simulink model "n2_linearized_system_control"  (R2023b)
settings: Solver=VariableStepAuto  StartTime=0.0  StopTime=3  RelTol=1e-3
values from neighbouring files (symbols this model uses):
  Alin = [0    -k/Jl + m*g*l*sin(x2_bar)/Jl                     0           k/Jl ... (first row only)    [collaborative_class_main.m]    (also in n0_collaborative_class_main.m)
  Blin = [0; 0; 1/Jm; 0]    [collaborative_class_main.m]    (also in n0_collaborative_class_main.m)
  dx_0 = [0;1;0;1]*0.1    [n0_collaborative_class_main.m]    (also in svc_robot.m)
  K = place(Alin, Blin, p)    [collaborative_class_main.m]    (also in n0_collaborative_class_main.m)
  K_H2_V = K_H2(:, 5)    [collaborative_class_main.m]    (also in n0_collaborative_class_main.m)
  K_H2_X = K_H2(:,1:4)    [collaborative_class_main.m]    (also in n0_collaborative_class_main.m)
  K_lqeta = K_lqe(:, 5)    [collaborative_class_main.m]    (also in n0_collaborative_class_main.m)
  K_lqx = K_lqe(:,1:4)    [collaborative_class_main.m]    (also in n0_collaborative_class_main.m)
  Kv = -K_ext(1, 5)    [collaborative_class_main.m]    (also in n0_collaborative_class_main.m)
  Kx = -K_ext(1, 1:4)    [collaborative_class_main.m]    (also in n0_collaborative_class_main.m)
  u_bar = m*g*l*cos(x2_bar)    [collaborative_class_main.m]    (also in n0_collaborative_class_main.m; svc_robot.m)
undefined symbols (not defined in the file or in its folder): K_lq
settings Model: Creator=teoma  LastModifiedBy=teoma

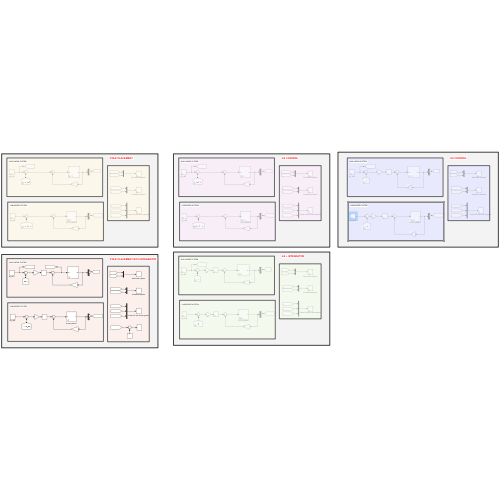
[thumbnail: Simulink's stored preview of the top-level diagram]
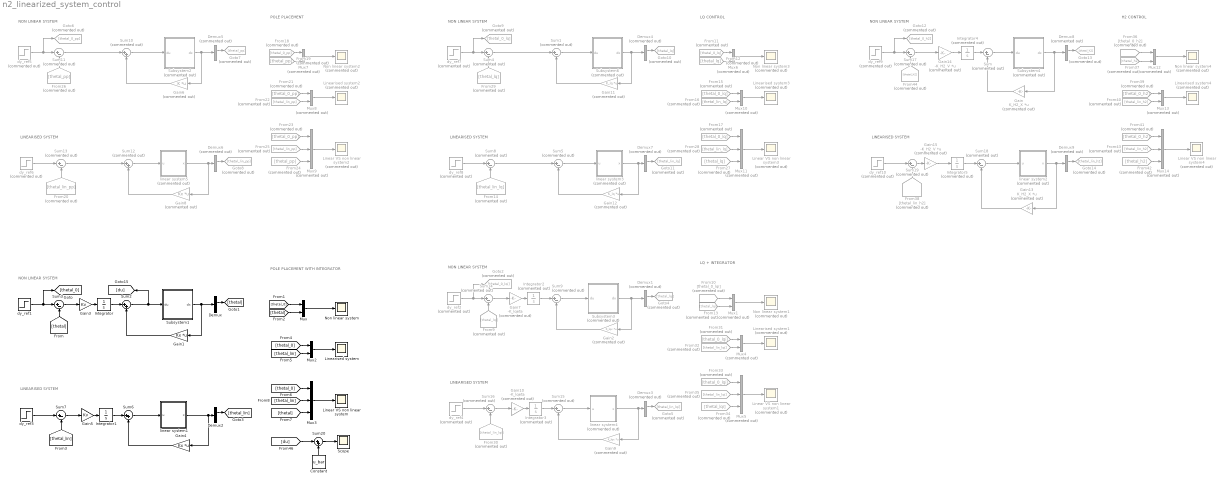
== system n2_linearized_system_control ==
  note: POLE PLACEMENT WITH INTEGRATOR
  note: NON LINEAR SYSTEM
  note: LINEARISED SYSTEM
  note: POLE PLACEMENT
  note: LINEARISED SYSTEM
  note: NON LINEAR SYSTEM
  note: NON LINEAR SYSTEM
  note: LQ CONTROL
  note: LINEARISED SYSTEM
  note: NON LINEAR SYSTEM
  note: LINEARISED SYSTEM
  note: LQ + INTEGRATOR
  note: LINEARISED SYSTEM
  note: H2 CONTROL
  note: NON LINEAR SYSTEM
  Constant : Constant  Value=u_bar
  Demux : Demux
  Demux{1,3..9} (8 alike) : Demux  Commented=on
  Demux2 : Demux
  From10 : From  Commented=on  GotoTag=thetal_0_lqi
  From11 : From  Commented=on  GotoTag=thetal_0_lq
  From12 : From  Commented=on  GotoTag=thetal_lq
  From13 : From  Commented=on  GotoTag=thetal_lqi
  From14 : From  Commented=on  GotoTag=thetal_lin_lq
  From15 : From  Commented=on  GotoTag=thetal_0_lq
  From16 : From  Commented=on  GotoTag=thetal_lin_lq
  From17 : From  Commented=on  GotoTag=thetal_0_lq
  From18 : From  Commented=on  GotoTag=thetal_0_pp
  From19 : From  Commented=on  GotoTag=thetal_pp
  From20 : From  Commented=on  GotoTag=thetal_lin_pp
  From21 : From  Commented=on  GotoTag=thetal_0_pp
  From22 : From  Commented=on  GotoTag=thetal_lin_pp
  From23 : From  Commented=on  GotoTag=thetal_0_pp
  From24 : From  Commented=on  GotoTag=thetal_pp
  From25 : From  Commented=on  GotoTag=thetal_lin_pp
  From26 : From  Commented=on  GotoTag=thetal_pp
  From27 : From  Commented=on  GotoTag=thetal_lq
  From28 : From  Commented=on  GotoTag=thetal_lin_lq
  From29 : From  Commented=on  GotoTag=thetal_lq
  From30 : From  Commented=on  GotoTag=thetal_lin_lqi
  From31 : From  Commented=on  GotoTag=thetal_0_lqi
  From32 : From  Commented=on  GotoTag=thetal_lin_lqi
  From33 : From  Commented=on  GotoTag=thetal_0_lqi
  From34 : From  Commented=on  GotoTag=thetal_lqi
  From35 : From  Commented=on  GotoTag=thetal_lin_lqi
  From36 : From  Commented=on  GotoTag=thetal_0_h2
  From37 : From  Commented=on  GotoTag=thetal_h2
  From38 : From  Commented=on  GotoTag=thetal_lin_h2
  From39 : From  Commented=on  GotoTag=thetal_0_h2
  From40 : From  Commented=on  GotoTag=thetal_lin_h2
  From41 : From  Commented=on  GotoTag=thetal_0_h2
  From42 : From  Commented=on  GotoTag=thetal_h2
  From43 : From  Commented=on  GotoTag=thetal_lin_h2
  From44 : From  Commented=on  GotoTag=thetal_h2
  From9 : From  Commented=on  GotoTag=thetal_lqi
  Gain : Gain  Commented=on  Gain=K_H2_X  Multiplication=Matrix(K*u) (u vector)
  Gain1 : Gain  Gain=Kx  Multiplication=Matrix(K*u) (u vector)
  Gain10 : Gain  Commented=on  Gain=-K_lqeta
  Gain11 : Gain  Commented=on  Gain=K_lq  Multiplication=Matrix(K*u) (u vector)
  Gain12 : Gain  Commented=on  Gain=K_lq  Multiplication=Matrix(K*u) (u vector)
  Gain13 : Gain  Commented=on  Gain=K_H2_X  Multiplication=Matrix(K*u) (u vector)
  Gain14 : Gain  Commented=on  Gain=-K_H2_V  Multiplication=Matrix(K*u) (u vector)
  Gain15 : Gain  Commented=on  Gain=-K_H2_V  Multiplication=Matrix(K*u) (u vector)
  Gain2 : Gain  Commented=on  Gain=K_lqx  Multiplication=Matrix(K*u) (u vector)
  Gain3 : Gain  Gain=Kv
  Gain4 : Gain  Gain=Kx  Multiplication=Matrix(K*u) (u vector)
  Gain5 : Gain  Gain=Kv
  Gain6 : Gain  Commented=on  Gain=K  Multiplication=Matrix(K*u) (u vector)
  Gain7 : Gain  Commented=on  Gain=-K_lqeta
  Gain8 : Gain  Commented=on  Gain=Kx  Multiplication=Matrix(K*u) (u vector)
  Gain9 : Gain  Commented=on  Gain=K_lqx  Multiplication=Matrix(K*u) (u vector)
  Goto10 : Goto  Commented=on  GotoTag=thetal_lq
  Goto11 : Goto  Commented=on  GotoTag=thetal_lin_lq
  Goto12 : Goto  Commented=on  GotoTag=thetal_0_h2
  Goto13 : Goto  Commented=on  GotoTag=thetal_h2
  Goto14 : Goto  Commented=on  GotoTag=thetal_lin_h2
  Goto2 : Goto  Commented=on  GotoTag=thetal_0_lqi
  Goto4 : Goto  Commented=on  GotoTag=thetal_lqi
  Goto5 : Goto  Commented=on  GotoTag=thetal_lin_lqi
  Goto6 : Goto  Commented=on  GotoTag=thetal_0_pp
  Goto7 : Goto  Commented=on  GotoTag=thetal_pp
  Goto8 : Goto  Commented=on  GotoTag=thetal_lin_pp
  Goto9 : Goto  Commented=on  GotoTag=thetal_0_lq
  Integrator : Integrator
  Integrator1 : Integrator
  Integrator{2..5} (4 alike) : Integrator  Commented=on
  Linear VS non linear system : Scope
  Linear VS non linear system{1..4} (4 alike) : Scope  Commented=on
  Linearised system : Scope
  Linearised system{1..4} (4 alike) : Scope  Commented=on
  Mux : Mux  Inputs=2
  Mux{1,4,6..8,10,12..13} (8 alike) : Mux  Commented=on  Inputs=2
  Mux{5,9,11,14} (4 alike) : Mux  Commented=on  Inputs=3
  Mux2 : Mux  Inputs=2
  Mux3 : Mux  Inputs=3
  Non linear system : Scope
  Non linear system{1..4} (4 alike) : Scope  Commented=on
  Scope : Scope
  Subsystem1 : Subsystem  mask{dx_0=dx_0}
      mask prompts: dx_0 "initial state"
  Subsystem2 : Subsystem  Commented=on  mask{dx_0=dx_0}
      mask prompts: dx_0 "initial state"
  Subsystem3 : Subsystem  Commented=on  mask{dx_0=dx_0}
      mask prompts: dx_0 "initial state"
  Subsystem4 : Subsystem  Commented=on  mask{dx_0=dx_0}
      mask prompts: dx_0 "initial state"
  Subsystem6 : Subsystem  Commented=on  mask{dx_0=dx_0}
      mask prompts: dx_0 "initial state"
  Sum{,1,4..5,8..9,11,13..19} (14 alike) : Sum  Commented=on  Inputs=|+-
  Sum10 : Sum  Commented=on  Inputs=|++
  Sum12 : Sum  Commented=on  Inputs=|++
  Sum2 : Sum  Inputs=|++
  Sum20 : Sum  Inputs=|++
  Sum3 : Sum  Inputs=|+-
  Sum6 : Sum  Inputs=|++
  Sum7 : Sum  Inputs=|+-
  dy_ref1 : Step  After=0.1  SampleTime=0
  dy_ref{2,4,9..10} (4 alike) : Step  Commented=on  Time=0  After=0.1  SampleTime=0
  dy_ref3 : Step  After=0.1  SampleTime=0
  dy_ref{5..8} (4 alike) : Step  Commented=on  After=0.1  SampleTime=0
  linear system1 : Subsystem  mask{dx_0=dx_0}
      mask prompts: dx_0 "initial state"
  linear system2 : Subsystem  Commented=on  mask{dx_0=dx_0}
      mask prompts: dx_0 "initial state"
  linear system3 : Subsystem  Commented=on  mask{dx_0=dx_0}
      mask prompts: dx_0 "initial state"
  linear system4 : Subsystem  Commented=on  mask{dx_0=dx_0}
      mask prompts: dx_0 "initial state"
  linear system5 : Subsystem  Commented=on  mask{dx_0=dx_0}
      mask prompts: dx_0 "initial state"
  wires:
  Subsystem1/1(dx) -> Gain1/1, Demux/1
  Sum2/1 -> [du], Subsystem1/1(du)
  Gain1/1 -> Sum2/2
  dy_ref1/1 -> [thetal_0], Sum3/1
  Mux/1 -> Non linear system/1
  Sum3/1 -> Gain3/1
  Gain3/1 -> Integrator/1
  Integrator/1 -> Sum2/1
  Demux/2 -> [thetal]
  [thetal] -> Sum3/2
  [thetal_0] -> Mux/1
  [thetal] -> Mux/2
  dy_ref3/1 -> Sum7/1
  Sum7/1 -> Gain5/1
  Sum6/1 -> linear system1/1(u)
  [thetal_lin] -> Mux2/2
  Gain4/1 -> Sum6/2
  Mux2/1 -> Linearised system/1
  Gain5/1 -> Integrator1/1
  Integrator1/1 -> Sum6/1
  [thetal_0] -> Mux2/1
  [thetal_lin] -> Sum7/2
  Demux2/2 -> [thetal_lin]
  linear system1/1(x) -> Gain4/1, Demux2/1
  [thetal_0] -> Mux3/1
  [thetal] -> Mux3/3
  [thetal_lin] -> Mux3/2
  Mux3/1 -> Linear VS non linear system/1
  Sum10/1 -> Subsystem2/1(du)
  Mux7/1 -> Non linear system2/1
  From21/1 -> Mux8/1
  From19/1 -> Mux7/2
  Gain6/1 -> Sum10/2
  Subsystem2/1(dx) -> Gain6/1, Demux5/1
  From23/1 -> Mux9/1
  Mux8/1 -> Linearised system2/1
  linear system5/1(x) -> Gain8/1, Demux6/1
  Demux5/2 -> Goto7/1
  From26/1 -> Sum11/2
  From18/1 -> Mux7/1
  Gain8/1 -> Sum12/2
  Demux6/2 -> Goto8/1
  From20/1 -> Sum13/2
  Mux9/1 -> Linear VS non linear system2/1
  dy_ref6/1 -> Sum13/1
  From22/1 -> Mux8/2
  From25/1 -> Mux9/2
  From24/1 -> Mux9/3
  dy_ref5/1 -> Goto6/1, Sum11/1
  Sum11/1 -> Sum10/1
  Sum13/1 -> Sum12/1
  From33/1 -> Mux5/1
  Sum8/1 -> Sum5/1
  From29/1 -> Sum4/2
  Subsystem6/1(dx) -> Gain11/1, Demux4/1
  Integrator3/1 -> Sum15/1
  From17/1 -> Mux11/1
  Sum1/1 -> Subsystem6/1(du)
  Mux1/1 -> Non linear system1/1
  From32/1 -> Mux4/2
  Mux10/1 -> Linearised system3/1
  Demux3/2 -> Goto5/1
  Demux7/2 -> Goto11/1
  From15/1 -> Mux10/1
  Demux1/2 -> Goto4/1
  Mux6/1 -> Non linear system3/1
  From14/1 -> Sum8/2
  From11/1 -> Mux6/1
  From27/1 -> Mux11/3
  Sum4/1 -> Sum1/1
  From31/1 -> Mux4/1
  Gain11/1 -> Sum1/2
  Sum15/1 -> linear system4/1(u)
  dy_ref2/1 -> Goto2/1, Sum14/1
  Gain7/1 -> Integrator2/1
  Gain2/1 -> Sum9/2
  From10/1 -> Mux1/1
  From12/1 -> Mux6/2
  Gain9/1 -> Sum15/2
  dy_ref4/1 -> Sum16/1
  Subsystem3/1(dx) -> Gain2/1, Demux1/1
  From35/1 -> Mux5/2
  Gain10/1 -> Integrator3/1
  Sum16/1 -> Gain10/1
  Sum5/1 -> linear system3/1(u)
  From9/1 -> Sum14/2
  dy_ref8/1 -> Sum8/1
  From13/1 -> Mux1/2
  linear system4/1(x) -> Gain9/1, Demux3/1
  Sum14/1 -> Gain7/1
  dy_ref7/1 -> Goto9/1, Sum4/1
  Mux4/1 -> Linearised system1/1
  Mux11/1 -> Linear VS non linear system3/1
  linear system3/1(x) -> Gain12/1, Demux7/1
  From16/1 -> Mux10/2
  From28/1 -> Mux11/2
  Sum9/1 -> Subsystem3/1(du)
  Mux5/1 -> Linear VS non linear system1/1
  Demux4/2 -> Goto10/1
  From30/1 -> Sum16/2
  Gain12/1 -> Sum5/2
  From34/1 -> Mux5/3
  Integrator2/1 -> Sum9/1
  From40/1 -> Mux13/2
  Demux9/2 -> Goto14/1
  From43/1 -> Mux14/2
  From38/1 -> Sum19/2
  From37/1 -> Mux12/2
  Mux12/1 -> Non linear system4/1
  From44/1 -> Sum17/2
  From42/1 -> Mux14/3
  dy_ref10/1 -> Sum19/1
  From36/1 -> Mux12/1
  Demux8/2 -> Goto13/1
  From39/1 -> Mux13/1
  Subsystem4/1(dx) -> Gain/1, Demux8/1
  dy_ref9/1 -> Goto12/1, Sum17/1
  From41/1 -> Mux14/1
  Mux14/1 -> Linear VS non linear system4/1
  linear system2/1(x) -> Gain13/1, Demux9/1
  Mux13/1 -> Linearised system4/1
  Gain/1 -> Sum/2
  Sum/1 -> Subsystem4/1(du)
  Sum18/1 -> linear system2/1(u)
  Gain13/1 -> Sum18/2
  Gain14/1 -> Integrator4/1
  Gain15/1 -> Integrator5/1
  Sum17/1 -> Gain14/1
  Integrator4/1 -> Sum/1
  Sum19/1 -> Gain15/1
  Integrator5/1 -> Sum18/1
  Sum20/1 -> Scope/1
  Constant/1 -> Sum20/2
  [du] -> Sum20/1
  Sum12/1 -> linear system5/1(u)

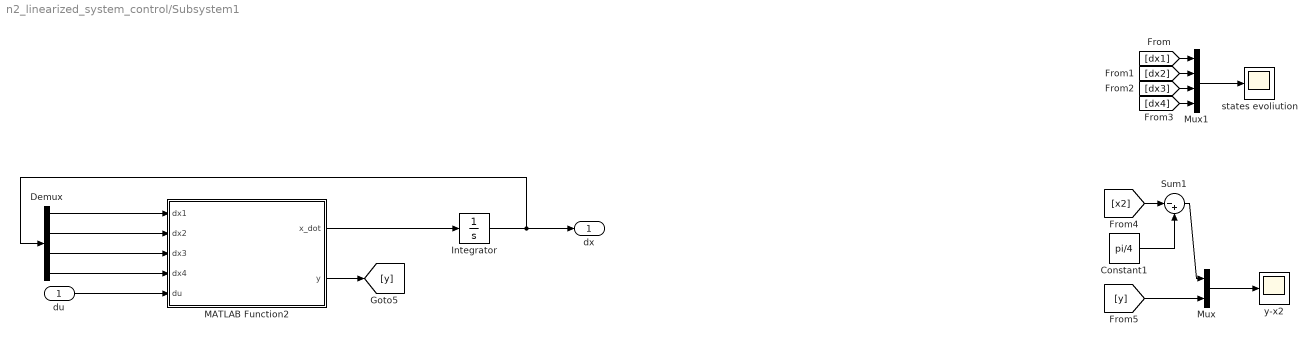
== system n2_linearized_system_control/Subsystem1 ==
  du : Inport
  Constant1 : Constant  Value=pi/4
  Demux : Demux
  Integrator : Integrator  InitialCondition=dx_0
  MATLAB Function2 : MATLAB Function  TreatAsAtomicUnit=on
  Mux : Mux  Inputs=2
  Mux1 : Mux
  Sum1 : Sum  Inputs=|-+
  "states evoliution " : Scope
  y-x2 : Scope
  dx : Outport
  wires:
  du/1 -> MATLAB Function2/5(du)
  MATLAB Function2/2(y) -> [y]
  Demux/1 -> MATLAB Function2/1(dx1)
  Demux/2 -> MATLAB Function2/2(dx2)
  Demux/3 -> MATLAB Function2/3(dx3)
  Demux/4 -> MATLAB Function2/4(dx4)
  MATLAB Function2/1(x_dot) -> Integrator/1
  Integrator/1 -> dx/1, Demux/1
  Mux/1 -> y-x2/1
  Sum1/1 -> Mux/1
  Constant1/1 -> Sum1/2
  [dx1] -> Mux1/1
  [dx2] -> Mux1/2
  [dx3] -> Mux1/3
  [dx4] -> Mux1/4
  Mux1/1 -> "states evoliution "/1
  [x2] -> Sum1/1
  [y] -> Mux/2

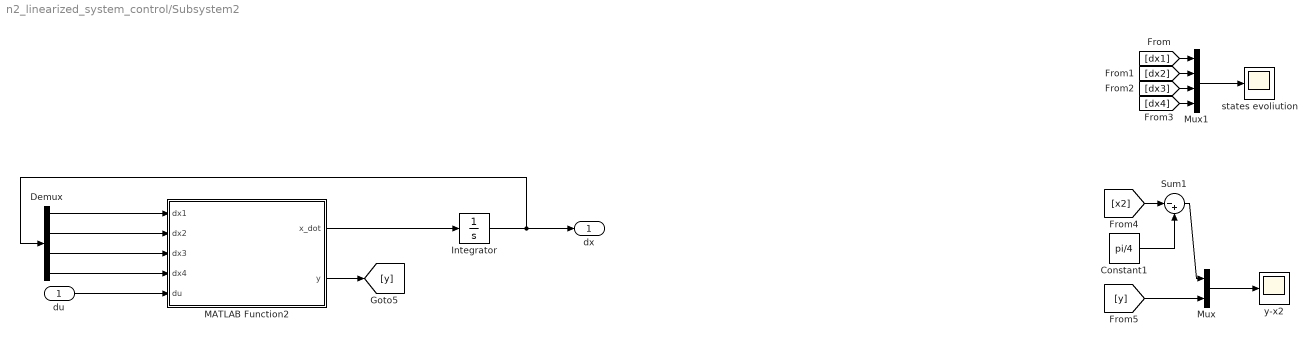
== system n2_linearized_system_control/Subsystem2 ==
  du : Inport
  Constant1 : Constant  Value=pi/4
  Demux : Demux
  Integrator : Integrator  InitialCondition=dx_0
  MATLAB Function2 : MATLAB Function  TreatAsAtomicUnit=on
  Mux : Mux  Inputs=2
  Mux1 : Mux
  Sum1 : Sum  Inputs=|-+
  "states evoliution " : Scope
  y-x2 : Scope
  dx : Outport
  wires:
  du/1 -> MATLAB Function2/5(du)
  MATLAB Function2/2(y) -> [y]
  Demux/1 -> MATLAB Function2/1(dx1)
  Demux/2 -> MATLAB Function2/2(dx2)
  Demux/3 -> MATLAB Function2/3(dx3)
  Demux/4 -> MATLAB Function2/4(dx4)
  MATLAB Function2/1(x_dot) -> Integrator/1
  Integrator/1 -> dx/1, Demux/1
  Mux/1 -> y-x2/1
  Sum1/1 -> Mux/1
  Constant1/1 -> Sum1/2
  [dx1] -> Mux1/1
  [dx2] -> Mux1/2
  [dx3] -> Mux1/3
  [dx4] -> Mux1/4
  Mux1/1 -> "states evoliution "/1
  [x2] -> Sum1/1
  [y] -> Mux/2

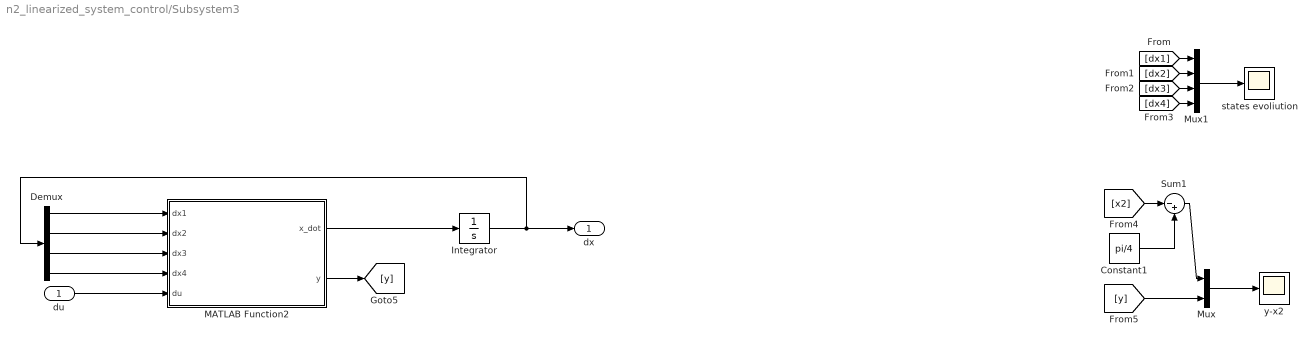
== system n2_linearized_system_control/Subsystem3 ==
  du : Inport
  Constant1 : Constant  Value=pi/4
  Demux : Demux
  Integrator : Integrator  InitialCondition=dx_0
  MATLAB Function2 : MATLAB Function  TreatAsAtomicUnit=on
  Mux : Mux  Inputs=2
  Mux1 : Mux
  Sum1 : Sum  Inputs=|-+
  "states evoliution " : Scope
  y-x2 : Scope
  dx : Outport
  wires:
  du/1 -> MATLAB Function2/5(du)
  MATLAB Function2/2(y) -> [y]
  Demux/1 -> MATLAB Function2/1(dx1)
  Demux/2 -> MATLAB Function2/2(dx2)
  Demux/3 -> MATLAB Function2/3(dx3)
  Demux/4 -> MATLAB Function2/4(dx4)
  MATLAB Function2/1(x_dot) -> Integrator/1
  Integrator/1 -> dx/1, Demux/1
  Mux/1 -> y-x2/1
  Sum1/1 -> Mux/1
  Constant1/1 -> Sum1/2
  [dx1] -> Mux1/1
  [dx2] -> Mux1/2
  [dx3] -> Mux1/3
  [dx4] -> Mux1/4
  Mux1/1 -> "states evoliution "/1
  [x2] -> Sum1/1
  [y] -> Mux/2

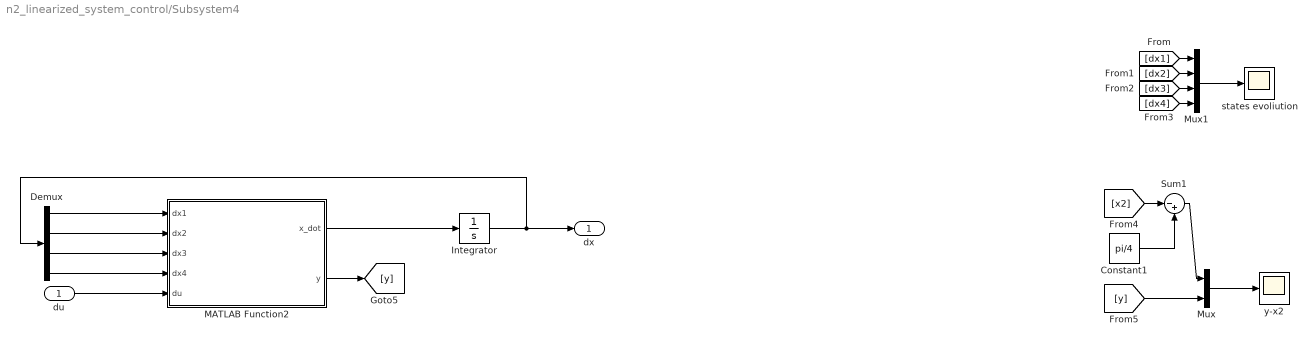
== system n2_linearized_system_control/Subsystem4 ==
  du : Inport
  Constant1 : Constant  Value=pi/4
  Demux : Demux
  Integrator : Integrator  InitialCondition=dx_0
  MATLAB Function2 : MATLAB Function  TreatAsAtomicUnit=on
  Mux : Mux  Inputs=2
  Mux1 : Mux
  Sum1 : Sum  Inputs=|-+
  "states evoliution " : Scope
  y-x2 : Scope
  dx : Outport
  wires:
  du/1 -> MATLAB Function2/5(du)
  MATLAB Function2/2(y) -> [y]
  Demux/1 -> MATLAB Function2/1(dx1)
  Demux/2 -> MATLAB Function2/2(dx2)
  Demux/3 -> MATLAB Function2/3(dx3)
  Demux/4 -> MATLAB Function2/4(dx4)
  MATLAB Function2/1(x_dot) -> Integrator/1
  Integrator/1 -> dx/1, Demux/1
  Mux/1 -> y-x2/1
  Sum1/1 -> Mux/1
  Constant1/1 -> Sum1/2
  [dx1] -> Mux1/1
  [dx2] -> Mux1/2
  [dx3] -> Mux1/3
  [dx4] -> Mux1/4
  Mux1/1 -> "states evoliution "/1
  [x2] -> Sum1/1
  [y] -> Mux/2

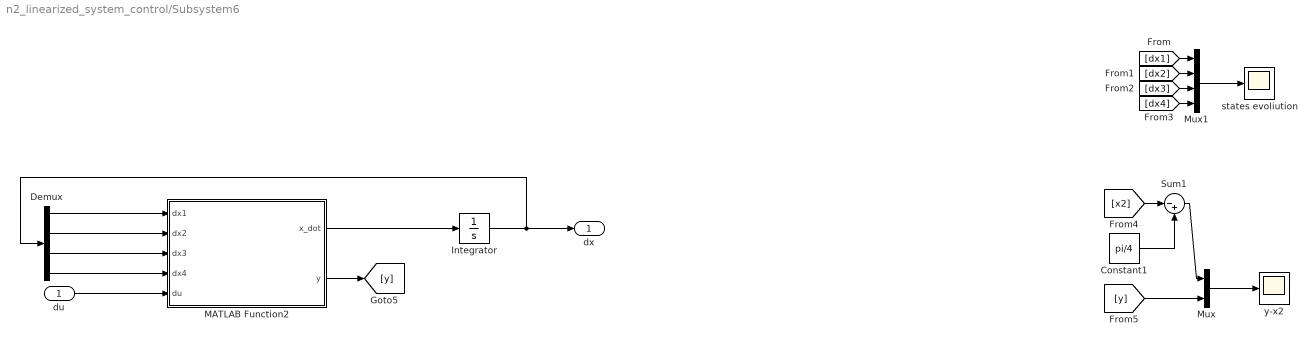
== system n2_linearized_system_control/Subsystem6 ==
  du : Inport
  Constant1 : Constant  Value=pi/4
  Demux : Demux
  Integrator : Integrator  InitialCondition=dx_0
  MATLAB Function2 : MATLAB Function  TreatAsAtomicUnit=on
  Mux : Mux  Inputs=2
  Mux1 : Mux
  Sum1 : Sum  Inputs=|-+
  "states evoliution " : Scope
  y-x2 : Scope
  dx : Outport
  wires:
  du/1 -> MATLAB Function2/5(du)
  MATLAB Function2/2(y) -> [y]
  Demux/1 -> MATLAB Function2/1(dx1)
  Demux/2 -> MATLAB Function2/2(dx2)
  Demux/3 -> MATLAB Function2/3(dx3)
  Demux/4 -> MATLAB Function2/4(dx4)
  MATLAB Function2/1(x_dot) -> Integrator/1
  Integrator/1 -> dx/1, Demux/1
  Mux/1 -> y-x2/1
  Sum1/1 -> Mux/1
  Constant1/1 -> Sum1/2
  [dx1] -> Mux1/1
  [dx2] -> Mux1/2
  [dx3] -> Mux1/3
  [dx4] -> Mux1/4
  Mux1/1 -> "states evoliution "/1
  [x2] -> Sum1/1
  [y] -> Mux/2

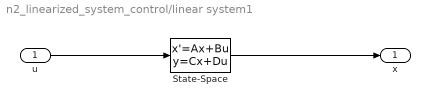
== system n2_linearized_system_control/linear system1 ==
  u : Inport
  State-Space : StateSpace  A=Alin  B=Blin  C=eye(4)  D=zeros(4,1)  InitialCondition=dx_0
  x : Outport
  wires:
  State-Space/1 -> x/1
  u/1 -> State-Space/1

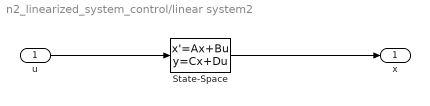
== system n2_linearized_system_control/linear system2 ==
  u : Inport
  State-Space : StateSpace  A=Alin  B=Blin  C=eye(4)  D=zeros(4,1)  InitialCondition=dx_0
  x : Outport
  wires:
  State-Space/1 -> x/1
  u/1 -> State-Space/1

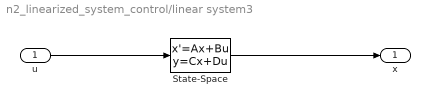
== system n2_linearized_system_control/linear system3 ==
  u : Inport
  State-Space : StateSpace  A=Alin  B=Blin  C=eye(4)  D=zeros(4,1)  InitialCondition=dx_0
  x : Outport
  wires:
  State-Space/1 -> x/1
  u/1 -> State-Space/1

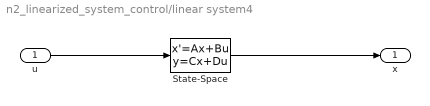
== system n2_linearized_system_control/linear system4 ==
  u : Inport
  State-Space : StateSpace  A=Alin  B=Blin  C=eye(4)  D=zeros(4,1)  InitialCondition=dx_0
  x : Outport
  wires:
  State-Space/1 -> x/1
  u/1 -> State-Space/1

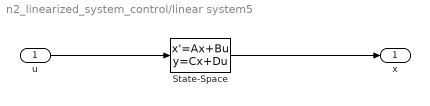
== system n2_linearized_system_control/linear system5 ==
  u : Inport
  State-Space : StateSpace  A=Alin  B=Blin  C=eye(4)  D=zeros(4,1)  InitialCondition=dx_0
  x : Outport
  wires:
  State-Space/1 -> x/1
  u/1 -> State-Space/1

== matlab function n2_linearized_system_control/Subsystem3/MATLAB Function2 ==
  data: dx1 input; dx2 input; dx3 input; dx4 input; du input; x_dot output; y output
function [x_dot, y]  = fcn(dx1,dx2,dx3,dx4, du)

k = 0.8;
Jm = 4e-4;
Jl= 4e-4;
Bm = 0.015;
Bl = 0;
m = 0.3;
l = 0.3;
g = 9.81;
x1_bar = 0;
x2_bar = pi/4;
x3_bar = 0;
x4_bar = m*g*l*cos(x2_bar)/k + x2_bar;
u_bar= m*g*l*cos(x2_bar);


x1_dot = -k/Jl*(dx2+x2_bar)-m*g*l/Jl*(cos(dx2+x2_bar))+k/Jl*(dx4+x4_bar);
x2_dot = dx1+x1_bar;
x3_dot = k/Jm*(dx2+x2_bar)-Bm/Jm*(dx3+x3_bar)-k/Jm*(dx4+x4_bar)+1/Jm*(du+u_bar);
x4_dot = dx3+x3_bar;
y = pi/4 - (dx2+x2_bar);

x_dot = zeros(1,4);
x_dot(1) = x1_dot;
x_dot(2) = x2_dot;
x_dot(3) = x3_dot;
x_dot(4) = x4_dot;

== matlab function n2_linearized_system_control/Subsystem2/MATLAB Function2 ==
  data: dx1 input; dx2 input; dx3 input; dx4 input; du input; x_dot output; y output
function [x_dot, y]  = fcn(dx1,dx2,dx3,dx4, du)

k = 0.8;
Jm = 4e-4;
Jl= 4e-4;
Bm = 0.015;
Bl = 0;
m = 0.3;
l = 0.3;
g = 9.81;
x1_bar = 0;
x2_bar = pi/4;
x3_bar = 0;
x4_bar = m*g*l*cos(x2_bar)/k + x2_bar;
u_bar= m*g*l*cos(x2_bar);


x1_dot = -k/Jl*(dx2+x2_bar)-m*g*l/Jl*(cos(dx2+x2_bar))+k/Jl*(dx4+x4_bar);
x2_dot = dx1+x1_bar;
x3_dot = k/Jm*(dx2+x2_bar)-Bm/Jm*(dx3+x3_bar)-k/Jm*(dx4+x4_bar)+1/Jm*(du+u_bar);
x4_dot = dx3+x3_bar;
y = pi/4 - (dx2+x2_bar);

x_dot = zeros(1,4);
x_dot(1) = x1_dot;
x_dot(2) = x2_dot;
x_dot(3) = x3_dot;
x_dot(4) = x4_dot;

== matlab function n2_linearized_system_control/Subsystem4/MATLAB Function2 ==
  data: dx1 input; dx2 input; dx3 input; dx4 input; du input; x_dot output; y output
function [x_dot, y]  = fcn(dx1,dx2,dx3,dx4, du)

k = 0.8;
Jm = 4e-4;
Jl= 4e-4;
Bm = 0.015;
Bl = 0;
m = 0.3;
l = 0.3;
g = 9.81;
x1_bar = 0;
x2_bar = pi/4;
x3_bar = 0;
x4_bar = m*g*l*cos(x2_bar)/k + x2_bar;
u_bar= m*g*l*cos(x2_bar);


x1_dot = -k/Jl*(dx2+x2_bar)-m*g*l/Jl*(cos(dx2+x2_bar))+k/Jl*(dx4+x4_bar);
x2_dot = dx1+x1_bar;
x3_dot = k/Jm*(dx2+x2_bar)-Bm/Jm*(dx3+x3_bar)-k/Jm*(dx4+x4_bar)+1/Jm*(du+u_bar);
x4_dot = dx3+x3_bar;
y = pi/4 - (dx2+x2_bar);

x_dot = zeros(1,4);
x_dot(1) = x1_dot;
x_dot(2) = x2_dot;
x_dot(3) = x3_dot;
x_dot(4) = x4_dot;

== matlab function n2_linearized_system_control/Subsystem1/MATLAB Function2 ==
  data: dx1 input; dx2 input; dx3 input; dx4 input; du input; x_dot output; y output
function [x_dot, y]  = fcn(dx1,dx2,dx3,dx4, du)

k = 0.8;
Jm = 4e-4;
Jl= 4e-4;
Bm = 0.015;
Bl = 0;
m = 0.3;
l = 0.3;
g = 9.81;
x1_bar = 0;
x2_bar = pi/4;
x3_bar = 0;
x4_bar = m*g*l*cos(x2_bar)/k + x2_bar;
u_bar= m*g*l*cos(x2_bar);


x1_dot = -k/Jl*(dx2+x2_bar)-m*g*l/Jl*(cos(dx2+x2_bar))+k/Jl*(dx4+x4_bar);
x2_dot = dx1+x1_bar;
x3_dot = k/Jm*(dx2+x2_bar)-Bm/Jm*(dx3+x3_bar)-k/Jm*(dx4+x4_bar)+1/Jm*(du+u_bar);
x4_dot = dx3+x3_bar;
y = pi/4 - (dx2+x2_bar);

x_dot = zeros(1,4);
x_dot(1) = x1_dot;
x_dot(2) = x2_dot;
x_dot(3) = x3_dot;
x_dot(4) = x4_dot;

== matlab function n2_linearized_system_control/Subsystem6/MATLAB Function2 ==
  data: dx1 input; dx2 input; dx3 input; dx4 input; du input; x_dot output; y output
function [x_dot, y]  = fcn(dx1,dx2,dx3,dx4, du)

k = 0.8;
Jm = 4e-4;
Jl= 4e-4;
Bm = 0.015;
Bl = 0;
m = 0.3;
l = 0.3;
g = 9.81;
x1_bar = 0;
x2_bar = pi/4;
x3_bar = 0;
x4_bar = m*g*l*cos(x2_bar)/k + x2_bar;
u_bar= m*g*l*cos(x2_bar);


x1_dot = -k/Jl*(dx2+x2_bar)-m*g*l/Jl*(cos(dx2+x2_bar))+k/Jl*(dx4+x4_bar);
x2_dot = dx1+x1_bar;
x3_dot = k/Jm*(dx2+x2_bar)-Bm/Jm*(dx3+x3_bar)-k/Jm*(dx4+x4_bar)+1/Jm*(du+u_bar);
x4_dot = dx3+x3_bar;
y = pi/4 - (dx2+x2_bar);

x_dot = zeros(1,4);
x_dot(1) = x1_dot;
x_dot(2) = x2_dot;
x_dot(3) = x3_dot;
x_dot(4) = x4_dot;
